simulink model "stateflow_2_logic_model"  (R2021b)
settings: Solver=VariableStepAuto  StartTime=0.0  StopTime=inf  RelTol=1e-3
settings Model: Creator=fredric  LastModifiedBy=fredric

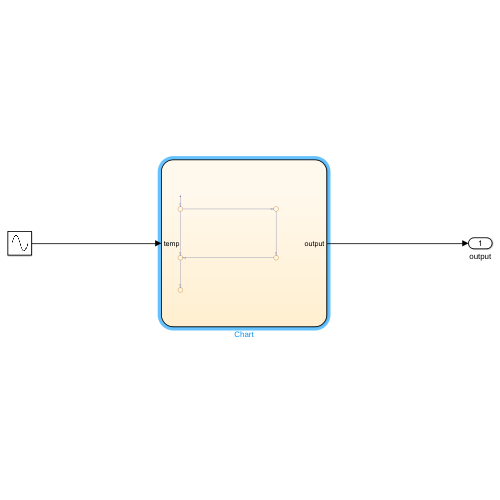
[thumbnail: Simulink's stored preview of the top-level diagram]
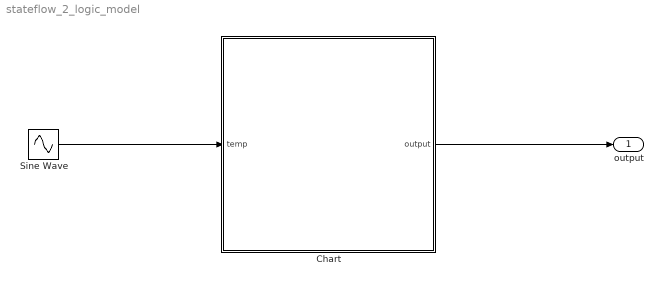
== system stateflow_2_logic_model ==
  Chart : Stateflow chart  TreatAsAtomicUnit=on
  Sine Wave : Sin  Amplitude=30  SampleTime=0
  output : Outport
  wires:
  Sine Wave/1 -> Chart/1(temp)
  Chart/1(output) -> output/1

== stateflow chart stateflow_2_logic_model/Chart ==
  (default) -> (junction 1)
  (junction 1) -> (junction 3) [order 1] : [temp > 26]
  (junction 1) -> (junction 7) [order 2] : {
      |
      |    output = 0;
      | }
  (junction 3) -> (junction 5) : {
      |
      |     output = -1;
      | }
  (junction 5) -> (junction 7)
  (junction 7) -> (junction 9)
  data: temp input; output output
